simulink model "Robot_Simulink_Discrete"  (R2018b)
settings: Solver=FixedStepDiscrete  StartTime=0.0  StopTime=Tt  FixedStep=Ts  RelTol=1e-3
values from neighbouring files (symbols this model uses):
  b = 0.25    [KF.m]    (also in Robot.m = 0.5)
  R_wl = 0.5    [KF.m]    (also in Robot.m = 0.35)
  R_wr = 0.5    [KF.m]    (also in Robot.m = 0.35)
  theta0 = pi/2    (= 1.57079632679)    [KF.m]    (also in Robot.m = 0.785398163397)
  Ts = 0.05    [KF.m]    (also in Robot.m = 0.01)
  u_wl = pi/2    (= 1.57079632679)    [KF.m]    (also in Robot.m)
  u_wr = pi/4    (= 0.785398163397)    [KF.m]    (also in Robot.m = 1.57079632679)
  x0 = 0    [KF.m]    (also in Robot.m)
  y0 = 0    [KF.m]    (also in Robot.m)
settings Model: Creator=Sergio  LastModifiedBy=Sergio

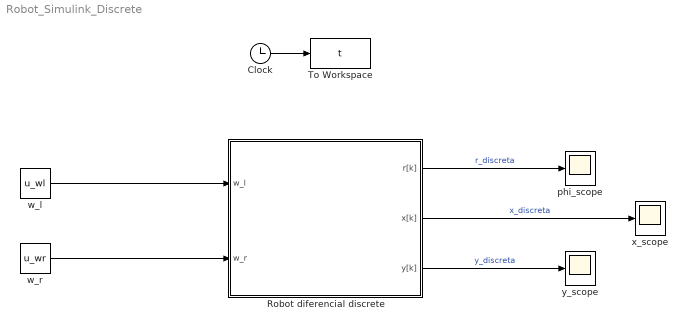
== system Robot_Simulink_Discrete ==
  Clock : Clock
  Robot diferencial discrete : Subsystem
      mask Display: image('D:\Máster Robótica y Automatización - msi\Asignaturas\Segundo cuatrimestre\Asignaturas\2.- Robots Móviles\2_ Material docente\Practicas\2018 -2019\Pr1 - Kalman Filter\Imagenes\Passive-Stability1.png');
  To Workspace : ToWorkspace  VariableName=t  SampleTime=-1
  phi_scope : Scope
  "w_l " : Constant  Value=u_wl
  "w_r " : Constant  Value=u_wr
  "x_scope " : Scope
  "y_scope " : Scope
  wires:
  Clock/1 -> To Workspace/1
  Robot diferencial discrete/2("x[k] ") -> "x_scope "/1  "x_discreta"
  Robot diferencial discrete/3("y[k] ") -> "y_scope "/1  "y_discreta"
  Robot diferencial discrete/1("r[k] ") -> phi_scope/1  "r_discreta"
  "w_l "/1 -> Robot diferencial discrete/1("w_l ")
  "w_r "/1 -> Robot diferencial discrete/2("w_r ")

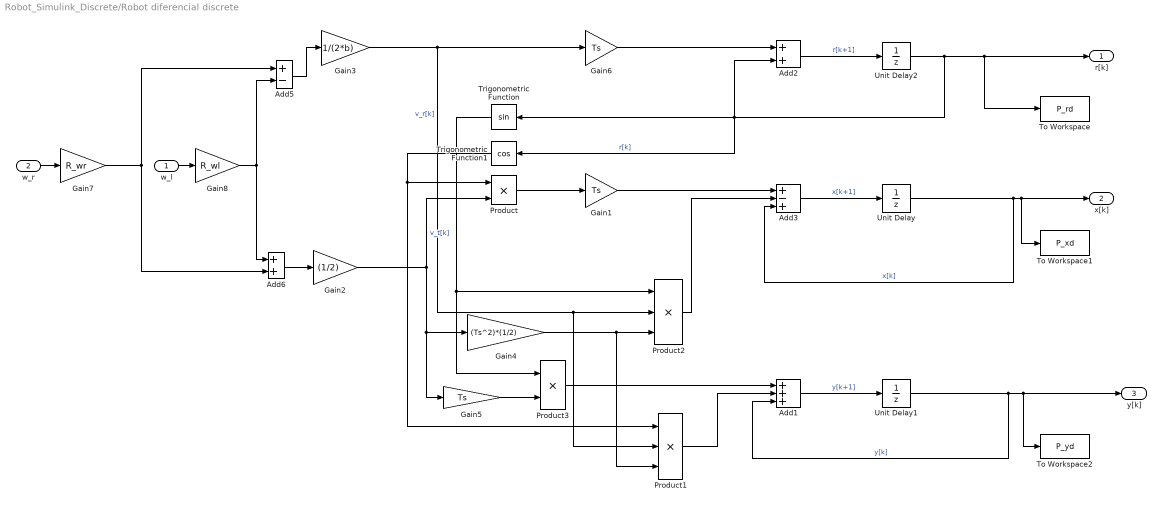
== system Robot_Simulink_Discrete/Robot diferencial discrete ==
  "w_l " : Inport
  "w_r " : Inport  Port=2
  Add1 : Sum  Inputs=+++
  Add2 : Sum
  Add3 : Sum  Inputs=+-+
  Add5 : Sum  Inputs=+-
  Add6 : Sum
  Gain1 : Gain  Gain=Ts
  Gain2 : Gain  Gain=(1/2)
  Gain3 : Gain  Gain=1/(2*b)
  Gain4 : Gain  Gain=(Ts^2)*(1/2)
  Gain5 : Gain  Gain=Ts
  Gain6 : Gain  Gain=Ts
  Gain7 : Gain  Gain=R_wr
  Gain8 : Gain  Gain=R_wl
  Product : Product
  Product1 : Product  Inputs=3
  Product2 : Product  Inputs=3
  Product3 : Product
  To Workspace : ToWorkspace  VariableName=P_rd  SampleTime=-1
  To Workspace1 : ToWorkspace  VariableName=P_xd  SampleTime=-1
  To Workspace2 : ToWorkspace  VariableName=P_yd  SampleTime=-1
  Trigonometric Function : Trigonometry
  Trigonometric Function1 : Trigonometry  Operator=cos
  Unit Delay : UnitDelay  InitialCondition=x0  SampleTime=Ts
  Unit Delay1 : UnitDelay  InitialCondition=y0  SampleTime=Ts
  Unit Delay2 : UnitDelay  InitialCondition=theta0  SampleTime=Ts
  "r[k] " : Outport
  "x[k] " : Outport  Port=2
  "y[k] " : Outport  Port=3
  wires:
  Add3/1 -> Unit Delay/1  "x[k+1]"
  Add1/1 -> Unit Delay1/1  "y[k+1]"
  Add2/1 -> Unit Delay2/1  "r[k+1]"
  Unit Delay/1 -> Add3/3, "x[k] "/1, To Workspace1/1  "x[k]"
  Unit Delay1/1 -> "y[k] "/1, To Workspace2/1, Add1/3  "y[k]"
  Add5/1 -> Gain3/1
  Unit Delay2/1 -> To Workspace/1, "r[k] "/1, Trigonometric Function1/1, Trigonometric Function/1, Add2/2  "r[k]"
  Add6/1 -> Gain2/1
  Product/1 -> Gain1/1
  Gain3/1 -> Product1/2, Product2/2, Gain6/1  "v_r[k]"
  Gain2/1 -> Gain5/1, Gain4/1, Product/2  "v_t[k]"
  Trigonometric Function1/1 -> Product/1, Product1/1
  Gain4/1 -> Product1/3, Product2/3
  Product2/1 -> Add3/2
  Trigonometric Function/1 -> Product2/1, Product3/1
  Gain5/1 -> Product3/2
  Product1/1 -> Add1/2
  "w_r "/1 -> Gain7/1
  Gain7/1 -> Add6/2, Add5/1
  "w_l "/1 -> Gain8/1
  Gain8/1 -> Add6/1, Add5/2
  Gain6/1 -> Add2/1
  Product3/1 -> Add1/1
  Gain1/1 -> Add3/1
